simulink model "ProyectoGlobal_AyCD_Cantu_LagoTejo_OPCUA"  (R2021a)
settings: Solver=ode23  StartTime=0.0  StopTime=inf  MinStep=1e-4
values from neighbouring files (symbols this model uses):
  a_hMax = 0.75    [Datos_ProyectoGlobal_AyCD_Cantu_LagoTejo.m]    (also in Datos_v18.m; PID_calculado.mat)
  a_tMax = 0.8    [Datos_ProyectoGlobal_AyCD_Cantu_LagoTejo.m]    (also in Datos_v18.m; PID_calculado.mat)
  b_cx = 1e6    (= 1000000)    [Datos_ProyectoGlobal_AyCD_Cantu_LagoTejo.m]    (also in Datos_v18.m; PID_calculado.mat)
  b_cy = 1e7    (= 10000000)    [Datos_ProyectoGlobal_AyCD_Cantu_LagoTejo.m]    (also in Datos_v18.m; PID_calculado.mat)
  b_eq_h = ((b_hd + b_hm*(i_h^2))*2/(r_hd^2))    (= 31004.4444444)    [Datos_ProyectoGlobal_AyCD_Cantu_LagoTejo.m]    (also in Datos_v18.m; PID_calculado.mat)
  b_eq_t = ((b_td + b_tm*(i_t^2))/(r_td^2))    (= 21607.2)    [Datos_ProyectoGlobal_AyCD_Cantu_LagoTejo.m]    (also in Datos_v18.m; PID_calculado.mat)
  b_hb = 1e8    (= 100000000)    [Datos_ProyectoGlobal_AyCD_Cantu_LagoTejo.m]    (also in Datos_v18.m; PID_calculado.mat)
  b_hEb = 2.2e9    (= 2200000000)    [Datos_ProyectoGlobal_AyCD_Cantu_LagoTejo.m]    (also in Datos_v18.m; PID_calculado.mat)
  b_t = 90    [Datos_ProyectoGlobal_AyCD_Cantu_LagoTejo.m]    (also in Datos_v18.m; PID_calculado.mat)
  b_tb = 5e6    (= 5000000)    [Datos_ProyectoGlobal_AyCD_Cantu_LagoTejo.m]    (also in Datos_v18.m; PID_calculado.mat)
  b_tw = 3e3    (= 3000)    [Datos_ProyectoGlobal_AyCD_Cantu_LagoTejo.m]    (also in Datos_v18.m; PID_calculado.mat)
  b_wu = 150    [Datos_ProyectoGlobal_AyCD_Cantu_LagoTejo.m]    (also in Datos_v18.m; PID_calculado.mat)
  bah = M_eq_h*n_h*omega_h    [PID_Izaje_B.m]    (also in PID_calculado.mat = 387555.555556)
  bat = M_eq_t*n_t*omega_t    [PID_Carro_B.m]    (also in PID_calculado.mat = 270090)
  CI_h = 5    [Datos_ProyectoGlobal_AyCD_Cantu_LagoTejo.m]    (also in Datos_v18.m; PID_calculado.mat)
  CI_t = -16.25    [Datos_ProyectoGlobal_AyCD_Cantu_LagoTejo.m]    (also in Datos_v18.m; PID_calculado.mat)
  g = 9.80665    [Datos_ProyectoGlobal_AyCD_Cantu_LagoTejo.m]    (also in Datos_v18.m; PID_calculado.mat)
  H_c = 2.5    [Datos_ProyectoGlobal_AyCD_Cantu_LagoTejo.m]    (also in Datos_v18.m; PID_calculado.mat)
  i_h = 22    [Datos_ProyectoGlobal_AyCD_Cantu_LagoTejo.m]    (also in Datos_v18.m; PID_calculado.mat)
  i_t = 30    [Datos_ProyectoGlobal_AyCD_Cantu_LagoTejo.m]    (also in Datos_v18.m; PID_calculado.mat)
  k_cy = 1.8e9    (= 1800000000)    [Datos_ProyectoGlobal_AyCD_Cantu_LagoTejo.m]    (also in Datos_v18.m; PID_calculado.mat)
  k_tw = 4.8e5    (= 480000)    [Datos_ProyectoGlobal_AyCD_Cantu_LagoTejo.m]    (also in Datos_v18.m; PID_calculado.mat)
  k_wu = 2.36e8    (= 236000000)    [Datos_ProyectoGlobal_AyCD_Cantu_LagoTejo.m]    (also in Datos_v18.m; PID_calculado.mat)
  Kd_bal = [-2.22044604925e-16 2.22044604925e-16 2.22044604925e-16 0 0 0 0 0 -2.22044604925e-16 0 2.22044604925e-16 -2.22044604925e-16 ... (296091 elements, 501x591)]    [Kp_Kd_balanceo.mat]    (also in PD_Balanceo.m = zeros(length(ML),length(L)))
  Kp_bal = [5.11381136401 5.1081388039 5.10248507909 5.09685008556 5.09123372013 5.08563588037 5.08005646467 5.07449537218 5.06895250283 5.06342775732 5.05792103709 5.05243224433 ... (296091 elements, 501x591)]    [Kp_Kd_balanceo.mat]    (also in PD_Balanceo.m = Kd_bal)
  ksah = M_eq_h*n_h*(omega_h^2)    [PID_Izaje_B.m]    (also in PID_calculado.mat = 922348.374575)
  ksat = M_eq_t*n_t*(omega_t^2)    [PID_Carro_B.m]    (also in PID_calculado.mat = 972648.108)
  ksiah = M_eq_h*n_h*(omega_h^3)    [PID_Izaje_B.m]    (also in PID_calculado.mat = 2195108.57705)
  ksiat = M_eq_t*n_t*(omega_t^3)    [PID_Carro_B.m]    (also in PID_calculado.mat = 3502700.36653)
  lim_xDer = 50    [Datos_ProyectoGlobal_AyCD_Cantu_LagoTejo.m]    (also in Datos_v18.m; PID_calculado.mat)
  lim_xDer_ult = 51    [Datos_ProyectoGlobal_AyCD_Cantu_LagoTejo.m]    (also in Datos_v18.m; PID_calculado.mat)
  lim_xIzq = -30    [Datos_ProyectoGlobal_AyCD_Cantu_LagoTejo.m]    (also in Datos_v18.m; PID_calculado.mat)
  lim_xIzq_ult = -31    [Datos_ProyectoGlobal_AyCD_Cantu_LagoTejo.m]    (also in Datos_v18.m; PID_calculado.mat)
  lim_yInf = -20    [Datos_ProyectoGlobal_AyCD_Cantu_LagoTejo.m]    (also in Datos_v18.m; PID_calculado.mat)
  lim_yInf_ult = -21    [Datos_ProyectoGlobal_AyCD_Cantu_LagoTejo.m]    (also in Datos_v18.m; PID_calculado.mat)
  lim_ySup = 40    [Datos_ProyectoGlobal_AyCD_Cantu_LagoTejo.m]    (also in Datos_v18.m; PID_calculado.mat)
  lim_ySup_ult = 41    [Datos_ProyectoGlobal_AyCD_Cantu_LagoTejo.m]    (also in Datos_v18.m; PID_calculado.mat)
  M_cMax = 50000    [Datos_ProyectoGlobal_AyCD_Cantu_LagoTejo.m]    (also in Datos_v18.m; PID_calculado.mat)
  M_cMin = 2000    [Datos_ProyectoGlobal_AyCD_Cantu_LagoTejo.m]    (also in Datos_v18.m; PID_calculado.mat)
  M_eq_h = (J_hd_hEb+J_hm_hb*i_h^2)*2/r_hd^2    (= 65137.7777778)    [Datos_ProyectoGlobal_AyCD_Cantu_LagoTejo.m]    (also in Datos_v18.m; PID_calculado.mat)
  M_eq_t = ((J_td + J_tm_tb*(i_t^2))/(r_td^2))    (= 30000)    [Datos_ProyectoGlobal_AyCD_Cantu_LagoTejo.m]    (also in Datos_v18.m; PID_calculado.mat)
  M_s = 15000    [Datos_ProyectoGlobal_AyCD_Cantu_LagoTejo.m]    (also in Datos_v18.m; PID_calculado.mat)
  M_t = 30000    [Datos_ProyectoGlobal_AyCD_Cantu_LagoTejo.m]    (also in Datos_v18.m; PID_calculado.mat)
  r_hd = 0.75    [Datos_ProyectoGlobal_AyCD_Cantu_LagoTejo.m]    (also in Datos_v18.m; PID_calculado.mat)
  r_td = 0.5    [Datos_ProyectoGlobal_AyCD_Cantu_LagoTejo.m]    (also in Datos_v18.m; PID_calculado.mat)
  T_hbMax = 5e4    (= 50000)    [Datos_ProyectoGlobal_AyCD_Cantu_LagoTejo.m]    (also in Datos_v18.m; PID_calculado.mat)
  T_hEbMax = 1.1e6    (= 1100000)    [Datos_ProyectoGlobal_AyCD_Cantu_LagoTejo.m]    (also in Datos_v18.m; PID_calculado.mat)
  T_hmMax = 2e4    (= 20000)    [Datos_ProyectoGlobal_AyCD_Cantu_LagoTejo.m]    (also in Datos_v18.m; PID_calculado.mat)
  T_tbMax = 5e3    (= 5000)    [Datos_ProyectoGlobal_AyCD_Cantu_LagoTejo.m]    (also in Datos_v18.m; PID_calculado.mat)
  T_tmMax = 3e3    (= 3000)    [Datos_ProyectoGlobal_AyCD_Cantu_LagoTejo.m]    (also in Datos_v18.m; PID_calculado.mat)
  tau_hm = 1e-3    (= 0.001)    [Datos_ProyectoGlobal_AyCD_Cantu_LagoTejo.m]    (also in Datos_v18.m; PID_calculado.mat)
  tau_tm = 1e-3    (= 0.001)    [Datos_ProyectoGlobal_AyCD_Cantu_LagoTejo.m]    (also in Datos_v18.m; PID_calculado.mat)
  v_hMax_0 = 3    [Datos_ProyectoGlobal_AyCD_Cantu_LagoTejo.m]    (also in Datos_v18.m; PID_calculado.mat)
  v_tMax = 4    [Datos_ProyectoGlobal_AyCD_Cantu_LagoTejo.m]    (also in Datos_v18.m; PID_calculado.mat)
  xc = [-28.75 -26.25 -23.75 -21.25 -18.75 -16.25 -13.75 -11.25 -8.75 -6.25 -3.75 -1.25 ... (32 elements, 1x32)]    [PID_calculado.mat]    (also in Perfil_Carga.m = -30+1.25:2.5:50-1.25)
  Y_t0 = 45    [Datos_ProyectoGlobal_AyCD_Cantu_LagoTejo.m]    (also in Datos_v18.m; PID_calculado.mat)
  yc = [0 0 0 2.5 0 2.5 0 2.5 0 0 0 0 ... (32 elements, 1x32)]    [PID_calculado.mat]    (also in Perfil_Carga.m = yc2)
undefined symbols (not defined in the file or in its folder): bcx, bcy, Cond_Ini_h, Cond_Ini_t, Kcy
libraries: simulink x13, opclib x3
(part 1 of 3)
settings Model: SimulationMode=accelerator  Creator=Maxi  LastModifiedBy=maxim
settings SolverCC: InitialStep=1e-3  MaxConsecutiveZCs=10000  MaxConsecutiveMinStep=10000000  ZeroCrossAlgorithm=Adaptive  AlgebraicLoopSolver=TrustRegion
settings DebuggingCC: AlgebraicLoopMsg=none  MaskedZcDiagnostic=none  IgnoredZcDiagnostic=none  SFUnusedDataAndEventsDiag=none  UnderSpecifiedDimensionMsg=warning
settings RTWCC: DLArmComputeVersion=20.02.1

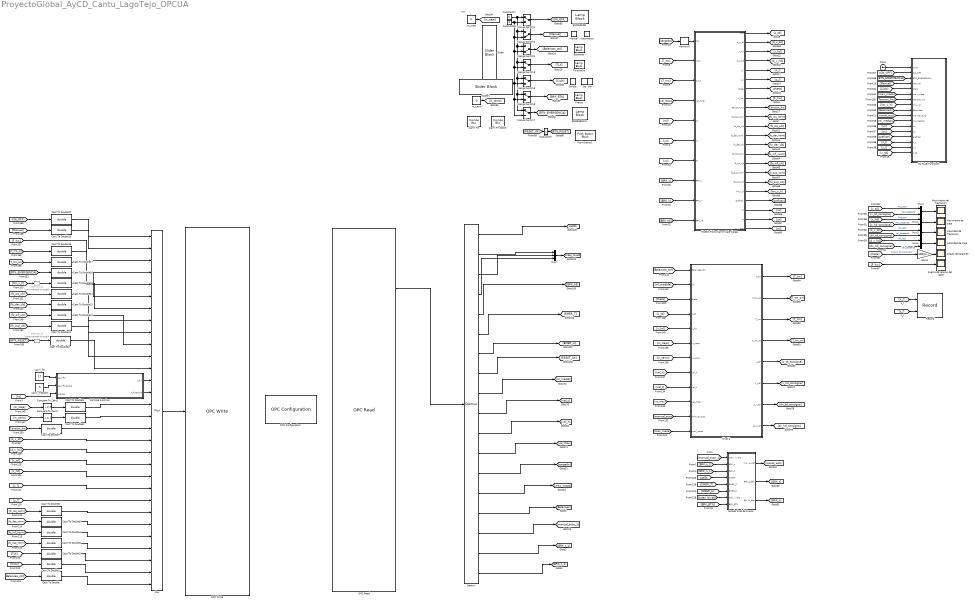
== system ProyectoGlobal_AyCD_Cantu_LagoTejo_OPCUA ==
  note: HMI
  "  Do" : LampBlock  LabelPosition=Hide
  Angulo de balanceo : Scope
  Automático : LampBlock  LabelPosition=Hide
  Balanceo : LampBlock  LabelPosition=Hide
  Carril Fin : ComboBox  LabelPosition=Hide  SelectedLabel=17
      settings: Values={{'1', '2', '3', '4', '5', '6', '7', '8', '9', '10', '11', '12', '13', '14', '15', '16', '17', '18'}, [1 2 3 4 5 6 7 8 9 10 11 12 13 14 15 16 17 18]}
  Carril Fin Doble : ComboBox  LabelPosition=Hide  SelectedLabel=5
      settings: Values={{'1', '2', '3', '4', '5', '6', '7', '8', '9', '10', '11', '12', '13', '14', '15', '16', '17', '18'}, [1 2 3 4 5 6 7 8 9 10 11 12 13 14 15 16 17 18]}
  Cast To Double{,1..20} (21 alike) : DataTypeConversion  OutDataTypeStr=double
  Clock : Clock
  Compare To Zero2 : simulink/Logic and Bit Operations/Compare To Zero  relop=~=  OutDataTypeStr=boolean
  Compare To Zero7 : simulink/Logic and Bit Operations/Compare To Zero  relop=~=  OutDataTypeStr=boolean
  Constant17 : Constant  Value=0
  Constant18 : Constant
  Demux : Demux  Outputs=18
  EMERGENCIA : LampBlock  LabelPosition=Hide
  ENCENDIDO : LampBlock  LabelPosition=Hide
  Estado Final de Frenos : Subsystem
  Frenos : LampBlock  LabelPosition=Hide
  Fuerza de tension del cable : Scope
  Gain3 : Gain  Gain=180/pi
  MATLAB Function : MATLAB Function  TreatAsAtomicUnit=on
  MATLAB Function1 : MATLAB Function  TreatAsAtomicUnit=on
  Manual : LampBlock  LabelPosition=Hide
  Manual Switch{1,3,5..7} (5 alike) : ManualSwitch
  Manual Switch2 : ManualSwitch  CurrentSetting=0
  Manual Switch4 : ManualSwitch  CurrentSetting=0
  Memory10 : Memory  Commented=through
  Memory12 : Memory  Commented=through
  Memory5 : Memory
  Modelo Fisico Carro-Izaje-Carga : Subsystem
  Movimiento de Izaje : Scope
  Movimiento de Traslacion : Scope
  Mux : Mux  Inputs=30
  Mux{1..4} (4 alike) : Mux  Inputs=2
  Mux7 : Mux  Inputs=3
  Nivel 2 : Subsystem
  OPC Configuration : opclib/OPC Configuration  opcServers=localhost/CoDeSys.OPC.DA/10  errMissingItems=Error  errReadWrite=Warn  errShutdown=Error  errRTViolation=Warn  rtEnable=on  speedup=1  showLatency=off  beingUsed=on
      settings: SourceProductBaseCode=OT
  OPC Read : opclib/OPC Read  serverHost=localhost  serverID=CoDeSys.OPC.DA  itemIDs=PLC1.Application.GVL.sistOK, PLC1.Application.GVL.manual_auto_N0, PLC1.Application.GVL.BRK_t_N0, PLC1.Application.GVL.BRK_h_N0, PLC1.Application.GVL.BRK_hE, PLC1.Application.GVL.EMER_t, PLC1.Application.GVL.EMER_h, PLC1.Application.GVL.RESET_OK, PLC1.Application.GVL.m_l_calc, PLC1.Application.GVL.vel_t, PLC1.Application.GVL.vel_h, PLC1.Application.GVL.vel_hMax, PLC1.Application.GVL.cargado, PLC1.Application.GVL.max_masa, PLC1.Application.GVL.Balanceo, PLC1.Application.GVL.manual_auto_N1, PLC1.Application.GVL.BRK_t_N1, PLC1.Application.GVL.BRK_h_N1  readMode=Synchronous (cache)  dataType=double  updateRate=0.5  showQual=on  showTS=on  tsMode=Seconds since start
      settings: SourceProductBaseCode=OT
  OPC Write : opclib/OPC Write  serverHost=localhost  serverID=CoDeSys.OPC.DA  itemIDs=PLC1.Application.GVL.ON_OFF, PLC1.Application.GVL.Manual, PLC1.Application.GVL.F_hw, PLC1.Application.GVL.T_hm_on, PLC1.Application.GVL.T_tm_on, PLC1.Application.GVL.BTN_EMERGENCIA, PLC1.Application.GVL.lim_v_h, PLC1.Application.GVL.fc_izq_ult, PLC1.Application.GVL.fc_der_ult, PLC1.Application.GVL.fc_inf_ult, PLC1.Application.GVL.fc_sup_ult, PLC1.Application.GVL.BTN_RESET, PLC1.Application.GVL.X_fin, PLC1.Application.GVL.X_finDoble, PLC1.Application.GVL.in_izaje_on, PLC1.Application.GVL.in_carro_on, PLC1.Application.GVL.Tension_hw, PLC1.Application.GVL.d_x_td, PLC1.Application.GVL.d_x_h, PLC1.Application.GVL.x_td, PLC1.Application.GVL.x_h, PLC1.Application.GVL.x_l, PLC1.Application.GVL.y_l, PLC1.Application.GVL.fc_izq_norm, PLC1.Application.GVL.fc_der_norm, PLC1.Application.GVL.fc_inf_norm, PLC1.Application.GVL.fc_sup_norm, PLC1.Application.GVL.TLK, PLC1.Application.GVL.Ciclo_Doble, PLC1.Application.GVL.Balanceo_ctrl  writeMode=Synchronous  updateRate=0
      settings: SourceProductBaseCode=OT
  Push Button1 : PushButtonBlock  ButtonText=RESET
  Record : Record  FileSettingsInternal="{\"entries\":[{\"content\":{\"excelSettings\":{\"content\":{},\"type\":\"Streamout.ExcelSettings\"}},\"type\":\"Streamout.FileSettingStorage\",\"uuid\":\"560a1c1a-7c8f-45a0-acac-2ad7503fa280\"}],\"packageUris\":[\"http://schema.mathworks.com/mf0/streamout_blocks/R2020a\"],\"version\":\"1.0\"}"  Layout=[1 1]  SignalsInternal="{\"entries\":[{\"content\":{\"signals\":[{\"content\":{\"blockPath\":[\"modelo_fisico_OPCUA/Record\"],\"channel\":[],\"dimensions\":[1],\"domain\":\"modelo_fisico_opcua/record\",\"lineColor\":\"#edb120\",\"plots\":[1],\"port\":1,\"sid\":[],\"signalID\":9,\"signalName\":\"x_l\"},\"type\":\"RecordBlkView.Signal\",\"uuid\":\"8ed411c4-7e14-4ae8-9e7a-a46f1e662131\"},{\"content\":{\"blockPath\":[\"modelo_fisico_OPCUA/Record\"],\"channel\":[],\"dimensions\":[1],\"domain\":\"modelo_fisico_opcua/record\",\"lineColor\":\"#7e2f8e\",\"plots\":[1],\"port\":2,\"sid\":[],\"signalID\":12,\"signalName\":\"y_l\"},\"type\":\"RecordBlkView.Signal\",\"uuid\":\"8d6d7a06-d56f-446f-a3f9-26de8d86f7e4\"},{\"content\":{\"blockPath\":[\"modelo_fisico_OPCUA/Record\"],\"channel\":[],\"dimensions\":[1,32],\"domain\":\"modelo_fisico_opcua/record\",\"hasChildren\":true,\"lineColor\":\"#77ac30\",\"plots\":[],\"port\":3,\"sid\":[],\"signalID\":15,\"signalName\":\"x_perfil\"},\"type\":\"RecordBlkView.Signal\",\"uuid\":\"b525593d-bc80-4908-881a-e4ffaca2af93\"},{\"content\":{\"blockPath\":[\"modelo_fisico_OPCUA/Record\"],\"channel\":[1,1],\"dimensions\":[1,32],\"domain\":\"modelo_fisico_opcua/record\",\"lineColor\":\"#4dbeee\",\"parentID\":15,\"plots\":[1],\"port\":3,\"sid\":[],\"signalID\":16,\"signalName\":\"x_perfil\"},\"type\":\"RecordBlkView.Signal\",\"uuid\":\"6a90bcad-4de9-4ccf-acf1-2125847e7892\"},{\"content\":{\"blockPath\":[\"modelo_fisico_OPCUA/Record\"],\"channel\":[1,2],\"dimensions\":[1,32],\"domain\":\"modelo_fisico_opcua/record\",\"lineColor\":\"#fe330a\",\"parentID\":15,\"plots\":[1],\"port\":3,\"sid\":[],\"signalID\":17,\"signalName\":\"x_perfil\"},\"type\":\"RecordBlkView.Signal\",\"uuid\":\"817aff20-781c-415f-a325-38912855be13\"},{\"content\":{\"blockPath\":[\"modelo_fisico_OPCUA/Record\"],\"channel\":[1,3],\"dimensions\":[1,32],\"domain\":\"modelo_fisico_opcua/record\",\"lineColor\":\"#22b573\",\"parentID\":15,\"plots\":[],\"port\":3,\"sid\":[],\"signalID\":18,\"signalName\":\"x_perfil\"},\"type\":\"RecordBlkView.Signal\",\"uuid\":\"17ad2ace-c9b0-4e9e-99ad-e43776de256b\"},{\"content\":{\"blockPath\":[\"modelo_fisico_OPCUA/Record\"],\"channel\":[1,4],\"dimensions\":[1,32],\"domain\":\"modelo_fisico_opcua/record\",\"lineColor\":\"#0072bd\",\"parentID\":15,\"plots\":[],\"port\":3,\"sid\":[],\"signalID\":19,\"signalName\":\"x_perfil\"},\"type\":\"RecordBlkView.Signal\",\"uuid\":\"ac0c197e-63a8-4e14-82ce-1afe2d8e9646\"},{\"content\":{\"blockPath\":[\"modelo_fisico_OPCUA/Record\"],\"channel\":[1,5],\"dimensions\":[1,32],\"domain\":\"modelo_fisico_opcua/record\",\"lineColor\":\"#d95319\",\"parentID\":15,\"plots\":[],\"port\":3,\"sid\":[],\"signalID\":20,\"signalName\":\"x_perfil\"},\"type\":\"RecordBlkView.Signal\",\"uuid\":\"b2dea709-1f7a-42de-b271-3351a57e50b4\"},{\"content\":{\"blockPath\":[\"modelo_fisico_OPCUA/Record\"],\"channel\":[1,6],\"dimensions\":[1,32],\"domain\":\"modelo_fisico_opcua/record\",\"lineColor\":\"#edb120\",\"parentID\":15,\"plots\":[],\"port\":3,\"sid\":[],\"signalID\":21,\"signalName\":\"x_perfil\"},\"type\":\"RecordBlkView.Signal\",\"uuid\":\"7040c539-c6c4-468b-b363-9105d925f59a\"},{\"content\":{\"blockPath\":[\"modelo_fisico_OPCUA/Record\"],\"channel\":[1,7],\"dimensions\":[1,32],\"domain\":\"modelo_fisico_opcua/record\",\"lineColor\":\"#7e2f8e\",\"parentID\":15,\"plots\":[],\"port\":3,\"sid\":[],\"signalID\":22,\"signalName\":\"x_perfil\"},\"type\":\"RecordBlkView.Signal\",\"uuid\":\"838ba2aa-2cf7-44e4-98a5-f5b176c14505\"},{\"content\":{\"blockPath\":[\"modelo_fisico_OPCUA/Record\"],\"channel\":[1,8],\"dimensions\":[1,32],\"domain\":\"modelo_fisico_opcua/record\",\"lineColor\":\"#77ac30\",\"parentID\":15,\"plots\":[],\"port\":3,\"sid\":[],\"signalID\":23,\"signalName\":\"x_perfil\"},\"type\":\"RecordBlkView.Signal\",\"uuid\":\"7f7327bd-a800-48a1-ae70-9791c063e958\"},{\"content\":{\"blockPath\":[\"modelo_fisico_OPCUA/Record\"],\"channel\":[1,9],\"dimensions\":[1,32],\"domain\":\"modelo_fisico_opcua/record\",\"lineColor\":\"#4dbeee\",\"parentID\":15,\"plots\":[],\"port\":3,\"sid\":[],\"signalID\":24,\"signalName\":\"x_perfil\"},\"type\":\"RecordBlkView.Signal\",\"uuid\":\"dc46df26-7320-47c5-a126-b064752e732b\"},{\"content\":{\"blockPath\":[\"modelo_fisico_OPCUA/Record\"],\"channel\":[1,10],\"dimensions\":[1,32],\"domain\":\"modelo_fisico_opcua/record\",\"lineColor\":\"#a2142f\",\"parentID\":15,\"plots\":[],\"port\":3,\"sid\":[],\"signalID\":25,\"signalName\":\"x_perfil\"},\"type\":\"RecordBlkView.Signal\",\"uuid\":\"56351981-dee7-481d-8877-4b0a4513273c\"},{\"content\":{\"blockPath\":[\"modelo_fisico_OPCUA/Record\"],\"channel\":[1,11],\"dimensions\":[1,32],\"domain\":\"modelo_fisico_opcua/record\",\"lineColor\":\"#139fff\",\"parentID\":15,\"plots\":[],\"port\":3,\"sid\":[],\"signalID\":26,\"signalName\":\"x_perfil\"},\"type\":\"RecordBlkView.Signal\",\"uuid\":\"c3cdab0a-47b4-4906-b085-8a2ff7353c31\"},{\"content\":{\"blockPath\":[\"modelo_fisico_OPCUA/Record\"],\"channel\":[1,12],\"dimensions\":[1,32],\"domain\":\"modelo_fisico_opcua/record\",\"lineColor\":\"#ff6929\",\"parentID\":15,\"plots\":[],\"port\":3,\"sid\":[],\"signalID\":27,\"signalName\":\"x_perfil\"},\"type\":\"RecordBlkView.Signal\",\"uuid\":\"92a94ddb-972e-4b54-aa74-364505e8725e\"},{\"content\":{\"blockPath\":[\"modelo_fisico_OPCUA/Record\"],\"channel\":[1,13],\"dimensions\":[1,32],\"domain\":\"modelo_fisico_opcua/record\",\"lineColor\":\"#b746ff\",\"parentID\":15,\"plots\":[],\"port\":3,\"sid\":[],\"signalID\":28,\"signalName\":\"x_perfil\"},\"type\":\"RecordBlkView.Signal\",\"uuid\":\"cd68ec88-6bbf-4001-a489-b4ac27c14d6a\"},{\"content\":{\"blockPath\":[\"modelo_fisico_OPCUA/Record\"],\"channel\":[1,14],\"dimensions\":[1,32],\"domain\":\"modelo_fisico_opcua/record\",\"lineColor\":\"#64d413\",\"parentID\":15,\"plots\":[],\"port\":3,\"sid\":[],\"signalID\":29,\"signalName\":\"x_perfil\"},\"type\":\"RecordBlkView.Signal\",\"uuid\":\"b6b0c035-5c4a-41dd-b6ed-91ecd091e6ef\"},{\"content\":{\"blockPath\":[\"modelo_fisico_OPCUA/Record\"],\"channel\":[1,15],\"dimensions\":[1,32],\"domain\":\"modelo_fisico_opcua/record\",\"lineColor\":\"#ff13a6\",\"parentID\":15,\"plots\":[],\"port\":3,\"sid\":[],\"signalID\":30,\"signalName\":\"x_perfil\"},\"type\":\"RecordBlkView.Signal\",\"uuid\":\"61be6124-0d23-485a-9b0c-6e628ce1c532\"},{\"content\":{\"blockPath\":[\"modelo_fisico_OPCUA/Record\"],\"channel\":[1,16],\"dimensions\":[1,32],\"domain\":\"modelo_fisico_opcua/record\",\"lineColor\":\"#fe330a\",\"parentID\":15,\"plots\":[],\"port\":3,\"sid\":[],\"signalID\":31,\"signalName\":\"x_perfil\"},\"type\":\"RecordBlkView.Signal\",\"uuid\":\"78409dcb-59a0-4571-a5b6-4d7693be06be\"},{\"content\":{\"blockPath\":[\"modelo_fisico_OPCUA/Record\"],\"channel\":[1,17],\"dimensions\":[1,32],\"domain\":\"modelo_fisico_opcua/record\",\"lineColor\":\"#22b573\",\"parentID\":15,\"plots\":[],\"port\":3,\"sid\":[],\"signalID\":32,\"signalName\":\"x_perfil\"},\"type\":\"RecordBlkView.Signal\",\"uuid\":\"40228b64-1439-4b88-8512-2e6e5e0a084f\"},{\"content\":{\"blockPath\":[\"modelo_fisico_OPCUA/Record\"],\"channel\":[1,18],\"dimensions\":[1,32],\"domain\":\"modelo_fisico_opcua/record\",\"lineColor\":\"#0072bd\",\"parentID\":15,\"plots\":[],\"port\":3,\"sid\":[],\"signalID\":33,\"signalName\":\"x_perfil\"},\"type\":\"RecordBlkView.Signal\",\"uuid\":\"d580995b-d659-4183-9c4a-5b8531b5410a\"},{\"content\":{\"blockPath\":[\"modelo_fisico_OPCUA/Record\"],\"channel\":[1,19],\"dimensions\":[1,32],\"domain\":\"modelo_fisico_opcua/record\",\"lineColor\":\"#d95319\",\"parentID\":15,\"plots\":[],\"port\":3,\"sid\":[],\"signalID\":34,\"signalName\":\"x_perfil\"},\"type\":\"RecordBlkView.Signal\",\"uuid\":\"362f2464-1207-4e23-923f-332f7297835c\"},{\"content\":{\"blockPath\":[\"modelo_fisico_OPCUA/Record\"],\"channel\":[1,20],\"dimensions\":[1,32],\"domain\":\"modelo_fisico_opcua/record\",\"lineColor\":\"#edb120\",\"parentID\":15,\"plots\":[],\"port\":3,\"sid\":[],\"signalID\":35,\"signalName\":\"x_perfil\"},\"type\":\"RecordBlkView.Signal\",\"uuid\":\"1b656f07-a23b-47d3-97d5-81b48fe59d30\"},{\"content\":{\"blockPath\":[\"modelo_fisico_OPCUA/Record\"],\"channel\":[1,21],\"dimensions\":[1,32],\"domain\":\"modelo_fisico_opcua/record\",\"lineColor\":\"#7e2f8e\",\"parentID\":15,\"plots\":[],\"port\":3,\"sid\":[],\"signalID\":36,\"signalName\":\"x_perfil\"},\"type\":\"RecordBlkView.Signal\",\"uuid\":\"41f2abfa-2a9f-43c7-8411-4d69c8cedf76\"},{\"content\":{\"blockPath\":[\"modelo_fisico_OPCUA/Record\"],\"channel\":[1,22],\"dimensions\":[1,32],\"domain\":\"modelo_fisico_opcua/record\",\"lineColor\":\"#77ac30\",\"parentID\":15,\"plots\":[],\"port\":3,\"sid\":[],\"signalID\":37,\"signalName\":\"x_perfil\"},\"type\":\"RecordBlkView.Signal\",\"uuid\":\"d0094ba1-20f3-4752-91cc-c8d7dc6f31e0\"},{\"content\":{\"blockPath\":[\"modelo_fisico_OPCUA/Record\"],\"channel\":[1,23],\"dimensions\":[1,32],\"domain\":\"modelo_fisico_opcua/record\",\"lineColor\":\"#4dbeee\",\"parentID\":15,\"plots\":[],\"port\":3,\"sid\":[],\"signalID\":38,\"signalName\":\"x_perfil\"},\"type\":\"RecordBlkView.Signal\",\"uuid\":\"7f1cb14b-d968-4eae-ae96-2eef0dcef1d2\"},{\"content\":{\"blockPath\":[\"modelo_fisico_OPCUA/Record\"],\"channel\":[1,24],\"dimensions\":[1,32],\"domain\":\"modelo_fisico_opcua/record\",\"lineColor\":\"#a2142f\",\"parentID\":15,\"plots\":[],\"port\":3,\"sid\":[],\"signalID\":39,\"signalName\":\"x_perfil\"},\"type\":\"RecordBlkView.Signal\",\"uuid\":\"a149b9b0-469b-4dee-b6a3-c3848182e778\"},{\"content\":{\"blockPath\":[\"modelo_fisico_OPCUA/Record\"],\"channel\":[1,25],\"dimensions\":[1,32],\"domain\":\"modelo_fisico_opcua/record\",\"lineColor\":\"#139fff\",\"parentID\":15,\"plots\":[],\"port\":3,\"sid\":[],\"signalID\":40,\"signalName\":\"x_perfil\"},\"type\":\"RecordBlkView.Signal\",\"uuid\":\"d2acd9f4-bf56-4995-9e9d-05fcbf398416\"},{\"content\":{\"blockPath\":[\"modelo_fisico_OPCUA/Record\"],\"channel\":[1,26],\"dimensions\":[1,32],\"domain\":\"modelo_fisico_opcua/record\",\"lineColor\":\"#ff6929\",\"parentID\":15,\"plots\":[],\"port\":3,\"sid\":[],\"signalID\":41,\"signalName\":\"x_perfil\"},\"type\":\"RecordBlkView.Signal\",\"uuid\":\"ec458ff0-2fe1-4e87-80ed-b9e014563081\"},{\"content\":{\"blockPath\":[\"modelo_fisico_OPCUA/Record\"],\"channel\":[1,27],\"dimensions\":[1,32],\"domain\":\"modelo_fisico_opcua/record\",\"lineColor\":\"#b746ff\",\"parentID\":15,\"plots\":[],\"port\":3,\"sid\":[],\"signalID\":42,\"signalName\":\"x_perfil\"},\"type\":\"RecordBlkView.Signal\",\"uuid\":\"6100f097-16d9-4f59-a052-147391a280cc\"},{\"content\":{\"blockPath\":[\"modelo_fisico_OPCUA/Record\"],\"channel\":[1,28],\"dimensions\":[1,32],\"domain\":\"modelo_fisico_opcua/record\",\"lineColor\":\"#64d413\",\"parentID\":15,\"plots\":[],\"port\":3,\"sid\":[],\"signalID\":43,\"signalName\":\"x_perfil\"},\"type\":\"RecordBlkView.Signal\",\"uuid\":\"f8afc42e-bebd-45e5-8773-ff8c2b40aedf\"},{\"content\":{\"blockPath\":[\"modelo_fisico_OPCUA/Record\"],\"channel\":[1,29],\"dimensions\":[1,32],\"domain\":\"modelo_fisico_opcua/record\",\"lineColor\":\"#ff13a6\",\"parentID\":15,\"plots\":[],\"port\":3,\"sid\":[],\"signalID\":44,\"signalName\":\"x_perfil\"},\"type\":\"RecordBlkView.Signal\",\"uuid\":\"3812678c-63e2-494a-8659-62fc09d91819\"},{\"content\":{\"blockPath\":[\"modelo_fisico_OPCUA/Record\"],\"channel\":[1,30],\"dimensions\":[1,32],\"domain\":\"modelo_fisico_opcua/record\",\"lineColor\":\"#fe330a\",\"parentID\":15,\"plots\":[],\"port\":3,\"sid\":[],\"signalID\":45,\"signalName\":\"x_perfil\"},\"type\":\"RecordBlkView.Signal\",\"uuid\":\"d3c92ddf-bef8-4ed9-8d40-50167eef2e7e\"},{\"content\":{\"blockPath\":[\"modelo_fisico_OPCUA/Record\"],\"channel\":[1,31],\"dimensions\":[1,32],\"domain\":\"modelo_fisico_opcua/record\",\"lineColor\":\"#22b573\",\"parentID\":15,\"plots\":[],\"port\":3,\"sid\":[],\"signalID\":46,\"signalName\":\"x_perfil\"},\"type\":\"RecordBlkView.Signal\",\"uuid\":\"6d648390-cc78-4833-a260-807b7828dc8a\"},{\"content\":{\"blockPath\":[\"modelo_fisico_OPCUA/Record\"],\"channel\":[1,32],\"dimensions\":[1,32],\"domain\":\"modelo_fisico_opcua/record\",\"lineColor\":\"#0072bd\",\"parentID\":15,\"plots\":[],\"port\":3,\"sid\":[],\"signalID\":47,\"signalName\":\"x_perfil\"},\"type\":\"RecordBlkView.Signal\",\"uuid\":\"42ae7673-7115-413a-868b-999b1065caa5\"},{\"content\":{\"blockPath\":[\"modelo_fisico_OPCUA/Record\"],\"channel\":[],\"dimensions\":[1,32],\"domain\":\"modelo_fisico_opcua/record\",\"hasChildren\":true,\"lineColor\":\"#a2142f\",\"plots\":[],\"port\":4,\"sid\":[],\"signalID\":82,\"signalName\":\"y_perfil\"},\"type\":\"RecordBlkView.Signal\",\"uuid\":\"d9f90962-6edd-4ec0-abe8-dd100a7f8a50\"},{\"content\":{\"blockPath\":[\"modelo_fisico_OPCUA/Record\"],\"channel\":[1,1],\"dimensions\":[1,32],\"domain\":\"modelo_fisico_opcua/record\",\"lineColor\":\"#139fff\",\"parentID\":82,\"plots\":[1],\"port\":4,\"sid\":[],\"signalID\":83,\"signalName\":\"y_perfil\"},\"type\":\"RecordBlkView.Signal\",\"uuid\":\"06b64a56-2c15-4519-8c10-7e671d1ef7ae\"},{\"content\":{\"blockPath\":[\"modelo_fisico_OPCUA/Record\"],\"channel\":[1,2],\"dimensions\":[1,32],\"domain\":\"modelo_fisico_opcua/record\",\"lineColor\":\"#d95319\",\"parentID\":82,\"plots\":[1],\"port\":4,\"sid\":[],\"signalID\":84,\"signalName\":\"y_perfil\"},\"type\":\"RecordBlkView.Signal\",\"uuid\":\"5fbd3c29-b525-4d08-ad80-dda292280f2b\"},{\"content\":{\"blockPath\":[\"modelo_fisico_OPCUA/Record\"],\"channel\":[1,3],\"dimensions\":[1,32],\"domain\":\"modelo_fisico_opcua/record\",\"lineColor\":\"#edb120\",\"parentID\":82,\"plots\":[],\"port\":4,\"sid\":[],\"signalID\":85,\"signalName\":\"y_perfil\"},\"type\":\"RecordBlkView.Signal\",\"uuid\":\"9489a3ba-12fc-47aa-bb2b-982bf65acc83\"},{\"content\":{\"blockPath\":[\"modelo_fisico_OPCUA/Record\"],\"channel\":[1,4],\"dimensions\":[1,32],\"domain\":\"modelo_fisico_opcua/record\",\"lineColor\":\"#7e2f8e\",\"parentID\":82,\"plots\":[],\"port\":4,\"sid\":[],\"signalID\":86,\"signalName\":\"y_perfil\"},\"type\":\"RecordBlkView.Signal\",\"uuid\":\"12117092-dea8-4a8e-a8b8-5264225c9133\"},{\"content\":{\"blockPath\":[\"modelo_fisico_OPCUA/Record\"],\"channel\":[1,5],\"dimensions\":[1,32],\"domain\":\"modelo_fisico_opcua/record\",\"lineColor\":\"#77ac30\",\"parentID\":82,\"plots\":[],\"port\":4,\"sid\":[],\"signalID\":87,\"signalName\":\"y_perfil\"},\"type\":\"RecordBlkView.Signal\",\"uuid\":\"3b763b01-e259-46f7-a043-73c60a8d4745\"},{\"content\":{\"blockPath\":[\"modelo_fisico_OPCUA/Record\"],\"channel\":[1,6],\"dimensions\":[1,32],\"domain\":\"modelo_fisico_opcua/record\",\"lineColor\":\"#4dbeee\",\"parentID\":82,\"plots\":[],\"port\":4,\"sid\":[],\"signalID\":88,\"signalName\":\"y_perfil\"},\"type\":\"RecordBlkView.Signal\",\"uuid\":\"3962a667-a6fe-4be6-9a61-c4fbe910ef5f\"},{\"content\":{\"blockPath\":[\"modelo_fisico_OPCUA/Record\"],\"channel\":[1,7],\"dimensions\":[1,32],\"domain\":\"modelo_fisico_opcua/record\",\"lineColor\":\"#a2142f\",\"parentID\":82,\"plots\":[],\"port\":4,\"sid\":[],\"signalID\":89,\"signalName\":\"y_perfil\"},\"type\":\"RecordBlkView.Signal\",\"uuid\":\"f27eb6c0-2ddc-4c38-a834-ebc399d71a7c\"},{\"content\":{\"blockPath\":[\"modelo_fisico_OPCUA/Record\"],\"channel\":[1,8],\"dimensions\":[1,32],\"domain\":\"modelo_fisico_opcua/record\",\"lineColor\":\"#139fff\",\"parentID\":82,\"plots\":[],\"port\":4,\"sid\":[],\"signalID\":90,\"signalName\":\"y_perfil\"},\"type\":\"RecordBlkView.Signal\",\"uuid\":\"c3f39b4b-3486-47ed-86bd-34da47593f3c\"},{\"content\":{\"blockPath\":[\"modelo_fisico_OPCUA/Record\"],\"channel\":[1,9],\"dimensions\":[1,32],\"domain\":\"modelo_fisico_opcua/record\",\"lineColor\":\"#ff6929\",\"parentID\":82,\"plots\":[],\"port\":4,\"sid\":[],\"signalID\":91,\"signalName\":\"y_perfil\"},\"type\":\"RecordBlkView.Signal\",\"uuid\":\"c598072b-d90f-4b6b-861e-e53c3de91533\"},{\"content\":{\"blockPath\":[\"modelo_fisico_OPCUA/Record\"],\"channel\":[1,10],\"dimensions\":[1,32],\"domain\":\"modelo_fisico_opcua/record\",\"lineColor\":\"#b746ff\",\"parentID\":82,\"plots\":[],\"port\":4,\"sid\":[],\"signalID\":92,\"signalName\":\"y_perfil\"},\"type\":\"RecordBlkView.Signal\",\"uuid\":\"2f3810d4-798f-48a7-bd67-4647fc5c2990\"},{\"content\":{\"blockPath\":[\"modelo_fisico_OPCUA/Record\"],\"channel\":[1,11],\"dimensions\":[1,32],\"domain\":\"modelo_fisico_opcua/record\",\"lineColor\":\"#64d413\",\"parentID\":82,\"plots\":[],\"port\":4,\"sid\":[],\"signalID\":93,\"signalName\":\"y_perfil\"},\"type\":\"RecordBlkView.Signal\",\"uuid\":\"c0af05f3-4e0f-441e-936b-860e4cc07fd4\"},{\"content\":{\"blockPath\":[\"modelo_fisico_OPCUA/Record\"],\"channel\":[1,12],\"dimensions\":[1,32],\"domain\":\"modelo_fisico_opcua/record\",\"lineColor\":\"#ff13a6\",\"parentID\":82,\"plots\":[],\"port\":4,\"sid\":[],\"signalID\":94,\"signalName\":\"y_perfil\"},\"type\":\"RecordBlkView.Signal\",\"uuid\":\"88dd4e19-5e1b-4e4e-a2b7-42439597bb32\"},{\"content\":{\"blockPath\":[\"modelo_fisico_OPCUA/Record\"],\"channel\":[1,13],\"dimensions\":[1,32],\"domain\":\"modelo_fisico_opcua/record\",\"lineColor\":\"#fe330a\",\"parentID\":82,\"plots\":[],\"port\":4,\"sid\":[],\"signalID\":95,\"signalName\":\"y_perfil\"},\"type\":\"RecordBlkView.Signal\",\"uuid\":\"472950a7-6a04-4c18-80e7-ec17a3b9bdd0\"},{\"content\":{\"blockPath\":[\"modelo_fisico_OPCUA/Record\"],\"channel\":[1,14],\"dimensions\":[1,32],\"domain\":\"modelo_fisico_opcua/record\",\"lineColor\":\"#22b573\",\"parentID\":82,\"plots\":[],\"port\":4,\"sid\":[],\"signalID\":96,\"signalName\":\"y_perfil\"},\"type\":\"RecordBlkView.Signal\",\"uuid\":\"b184d62d-1ce3-431c-818b-dfbc37fdbd4b\"},{\"content\":{\"blockPath\":[\"modelo_fisico_OPCUA/Record\"],\"channel\":[1,15],\"dimensions\":[1,32],\"domain\":\"modelo_fisico_opcua/record\",\"lineColor\":\"#0072bd\",\"parentID\":82,\"plots\":[],\"port\":4,\"sid\":[],\"signalID\":97,\"signalName\":\"y_perfil\"},\"type\":\"RecordBlkView.Signal\",\"uuid\":\"0fc82469-3e7a-4fd0-b72c-a38c6d423a6c\"},{\"content\":{\"blockPath\":[\"modelo_fisico_OPCUA/Record\"],\"channel\":[1,16],\"dimensions\":[1,32],\"domain\":\"modelo_fisico_opcua/record\",\"lineColor\":\"#d95319\",\"parentID\":82,\"plots\":[],\"port\":4,\"sid\":[],\"signalID\":98,\"signalName\":\"y_perfil\"},\"type\":\"RecordBlkView.Signal\",\"uuid\":\"26e3f7df-eb6c-47a6-ab40-ed8246f77387\"},{\"content\":{\"blockPath\":[\"modelo_fisico_OPCUA/Record\"],\"channel\":[1,17],\"dimensions\":[1,32],\"domain\":\"modelo_fisico_opcua/record\",\"lineColor\":\"#edb120\",\"parentID\":82,\"plots\":[],\"port\":4,\"sid\":[],\"signalID\":99,\"signalName\":\"y_perfil\"},\"type\":\"RecordBlkView.Signal\",\"uuid\":\"6c2c651d-418c-4fad-9cdc-7fdd0a0661a9\"},{\"content\":{\"blockPath\":[\"modelo_fisico_OPCUA/Record\"],\"channel\":[1,18],\"dimensions\":[1,32],\"domain\":\"modelo_fisico_opcua/record\",\"lineColor\":\"#7e2f8e\",\"parentID\":82,\"plots\":[],\"port\":4,\"sid\":[],\"signalID\":100,\"signalName\":\"y_perfil\"},\"type\":\"RecordBlkView.Signal\",\"uuid\":\"39474529-1a78-4fea-8b0b-9c9e9ee94a7e\"},{\"content\":{\"blockPath\":[\"modelo_fisico_OPCUA/Record\"],\"channel\":[1,19],\"dimensions\":[1,32],\"domain\":\"modelo_fisico_opcua/record\",\"lineColor\":\"#77ac30\",\"parentID\":82,\"plots\":[],\"port\":4,\"sid\":[],\"signalID\":101,\"signalName\":\"y_perfil\"},\"type\":\"RecordBlkView.Signal\",\"uuid\":\"7a3eb810-c178-4b33-8a1f-4ec4e8076906\"},{\"content\":{\"blockPath\":[\"modelo_fisico_OPCUA/Record\"],\"channel\":[1,20],\"dimensions\":[1,32],\"domain\":\"modelo_fisico_opcua/record\",\"lineColor\":\"#4dbeee\",\"parentID\":82,\"plots\":[1],\"port\":4,\"sid\":[],\"signalID\":102,\"signalName\":\"y_perfil\"},\"type\":\"RecordBlkView.Signal\",\"uuid\":\"773da45e-66fe-47bd-a564-c46eab3ad99f\"},{\"content\":{\"blockPath\":[\"modelo_fisico_OPCUA/Record\"],\"channel\":[1,21],\"dimensions\":[1,32],\"domain\":\"modelo_fisico_opcua/record\",\"lineColor\":\"#a2142f\",\"parentID\":82,\"plots\":[],\"port\":4,\"sid\":[],\"signalID\":103,\"signalName\":\"y_perfil\"},\"type\":\"RecordBlkView.Signal\",\"uuid\":\"1dcfc39f-9a11-4080-b0f4-1fc0b58cea96\"},{\"content\":{\"blockPath\":[\"modelo_fisico_OPCUA/Record\"],\"channel\":[1,22],\"dimensions\":[1,32],\"domain\":\"modelo_fisico_opcua/record\",\"lineColor\":\"#139fff\",\"parentID\":82,\"plots\":[],\"port\":4,\"sid\":[],\"signalID\":104,\"signalName\":\"y_perfil\"},\"type\":\"RecordBlkView.Signal\",\"uuid\":\"f55c5bef-511d-42d3-8889-be6042b26dfc\"},{\"content\":{\"blockPath\":[\"modelo_fisico_OPCUA/Record\"],\"channel\":[1,23],\"dimensions\":[1,32],\"domain\":\"modelo_fisico_opcua/record\",\"lineColor\":\"#ff6929\",\"parentID\":82,\"plots\":[],\"port\":4,\"sid\":[],\"signalID\":105,\"signalName\":\"y_perfil\"},\"type\":\"RecordBlkView.Signal\",\"uuid\":\"d588e2e1-5be1-40e5-af04-17a768d86c25\"},{\"content\":{\"blockPath\":[\"modelo_fisico_OPCUA/Record\"],\"channel\":[1,24],\"dimensions\":[1,32],\"domain\":\"modelo_fisico_opcua/record\",\"lineColor\":\"#b746ff\",\"parentID\":82,\"plots\":[],\"port\":4,\"sid\":[],\"signalID\":106,\"signalName\":\"y_perfil\"},\"type\":\"RecordBlkView.Signal\",\"uuid\":\"1561de11-5b82-49d1-9191-95153afd54cd\"},{\"content\":{\"blockPath\":[\"modelo_fisico_OPCUA/Record\"],\"channel\":[1,25],\"dimensions\":[1,32],\"domain\":\"modelo_fisico_opcua/record\",\"lineColor\":\"#64d413\",\"parentID\":82,\"plots\":[],\"port\":4,\"sid\":[],\"signalID\":107,\"signalName\":\"y_perfil\"},\"type\":\"RecordBlkView.Signal\",\"uuid\":\"501b56e5-fd3e-44d6-888f-617d8f2d249b\"},{\"content\":{\"blockPath\":[\"modelo_fisico_OPCUA/Record\"],\"channel\":[1,26],\"dimensions\":[1,32],\"domain\":\"modelo_fisico_opcua/record\",\"lineColor\":\"#ff13a6\",\"parentID\":82,\"plots\":[],\"port\":4,\"sid\":[],\"signalID\":108,\"signalName\":\"y_perfil\"},\"type\":\"RecordBlkView.Signal\",\"uuid\":\"3e59a2a9-a453-4f8e-af2b-13bfae1fb800\"},{\"content\":{\"blockPath\":[\"modelo_fisico_OPCUA/Record\"],\"channel\":[1,27],\"dimensions\":[1,32],\"domain\":\"modelo_fisico_opcua/record\",\"lineColor\":\"#fe330a\",\"parentID\":82,\"plots\":[],\"port\":4,\"sid\":[],\"signalID\":109,\"signalName\":\"y_perfil\"},\"type\":\"RecordBlkView.Signal\",\"uuid\":\"20d970d0-001e-4ddb-9f83-eed95db052ac\"},{\"content\":{\"blockPath\":[\"modelo_fisico_OPCUA/Record\"],\"channel\":[1,28],\"dimensions\":[1,32],\"domain\":\"modelo_fisico_opcua/record\",\"lineColor\":\"#22b573\",\"parentID\":82,\"plots\":[],\"port\":4,\"sid\":[],\"signalID\":110,\"signalName\":\"y_perfil\"},\"type\":\"RecordBlkView.Signal\",\"uuid\":\"171f34ef-737d-4a6b-adf4-5d8f884fe41d\"},{\"content\":{\"blockPath\":[\"modelo_fisico_OPCUA/Record\"],\"channel\":[1,29],\"dimensions\":[1,32],\"domain\":\"modelo_fisico_opcua/record\",\"lineColor\":\"#0072bd\",\"parentID\":82,\"plots\":[],\"port\":4,\"sid\":[],\"signalID\":111,\"signalName\":\"y_perfil\"},\"type\":\"RecordBlkView.Signal\",\"uuid\":\"f3cb6566-f680-4ede-b051-01350acaee5a\"},{\"content\":{\"blockPath\":[\"modelo_fisico_OPCUA/Record\"],\"channel\":[1,30],\"dimensions\":[1,32],\"domain\":\"modelo_fisico_opcua/record\",\"lineColor\":\"#d95319\",\"parentID\":82,\"plots\":[],\"port\":4,\"sid\":[],\"signalID\":112,\"signalName\":\"y_perfil\"},\"type\":\"RecordBlkView.Signal\",\"uuid\":\"e8776949-ef5e-4cff-8faf-37942e886e98\"},{\"content\":{\"blockPath\":[\"modelo_fisico_OPCUA/Record\"],\"channel\":[1,31],\"dimensions\":[1,32],\"domain\":\"modelo_fisico_opcua/record\",\"lineColor\":\"#edb120\",\"parentID\":82,\"plots\":[],\"port\":4,\"sid\":[],\"signalID\":113,\"signalName\":\"y_perfil\"},\"type\":\"RecordBlkView.Signal\",\"uuid\":\"1128a5de-0e88-454c-894a-b4c1c6e755a8\"},{\"content\":{\"blockPath\":[\"modelo_fisico_OPCUA/Record\"],\"channel\":[1,32],\"dimensions\":[1,32],\"domain\":\"modelo_fisico_opcua/record\",\"lineColor\":\"#7e2f8e\",\"parentID\":82,\"plots\":[],\"port\":4,\"sid\":[],\"signalID\":114,\"signalName\":\"y_perfil\"},\"type\":\"RecordBlkView.Signal\",\"uuid\":\"9fc86ab6-6c65-4a13-aef2-e178943432fa\"}]},\"type\":\"RecordBlkView.InputSignals\",\"uuid\":\"5fdf6d25-6721-45dd-a674-a9c5b544710a\"}],\"packageUris\":[\"http://schema.mathworks.com/mf0/streamout_blocks/R2020a\"],\"version\":\"1.0\"}"  VisualizationBindings="{\"xyplotplugin\":{\"info\":[{\"series\":[{\"bindingParametersList\":[{\"parameter\":\"X-Axis\",\"signalID\":9,\"signalName\":\"x_l\"},{\"parameter\":\"Y-Axis\",\"signalID\":12,\"signalName\":\"y_l\"}],\"seriesID\":213},{\"bindingParametersList\":[{\"parameter\":\"X-Axis\",\"signalID\":16,\"signalName\":\"x_perfil(1,1)\"},{\"parameter\":\"Y-Axis\",\"signalID\":83,\"signalName\":\"y_perfil(1,1)\"}],\"seriesID\":320},{\"bindingParametersList\":[{\"parameter\":\"X-Axis\",\"signalID\":17,\"signalName\":\"x_perfil(1,2)\"},{\"parameter\":\"Y-Axis\",\"signalID\":84,\"signalName\":\"y_perfil(1,2)\"}],\"seriesID\":639},{\"bindingParametersList\":[{\"parameter\":\"Y-Axis\",\"signalID\":102,\"signalName\":\"y_perfil(1,20)\"},{\"parameter\":\"X-Axis\",\"signalID\":102,\"signalName\":\"y_perfil(1,20)\"}],\"seriesID\":767}],\"subplotID\":1}]}}"
  Simple : LampBlock  LabelPosition=Hide
  Slider : SliderBlock  ScaleMin=-3  ScaleMax=3  TickInterval=1
  Slider1 : SliderBlock  ScaleMin=-4  ScaleMax=+4  TickInterval=1
  Subsystem : Subsystem
  Twistlocks : LampBlock  LabelPosition=Hide
  Velocidad de Izaje : Scope
  Velocidad de Traslacion : Scope
  "ble   " : LampBlock  LabelPosition=Hide
  carril_fin : Constant  Value=17
  carril_finDoble : Constant  Value=5
  in_carro : Constant  Value=0
  in_izaje : Constant  Value=0
  tag scope: Orden_Nivel0=global, sistOK=global
  wires:
  Modelo Fisico Carro-Izaje-Carga/1(x_td) -> [x_td]
  Modelo Fisico Carro-Izaje-Carga/3(x_hd) -> [x_hd]
  Modelo Fisico Carro-Izaje-Carga/7(theta) -> [theta]
  [yc] -> Modelo Fisico Carro-Izaje-Carga/6(Yc)
  Modelo Fisico Carro-Izaje-Carga/5(x_l) -> [x_l]
  Modelo Fisico Carro-Izaje-Carga/6(y_l) -> [y_l]
  Modelo Fisico Carro-Izaje-Carga/8(F_hw) -> [F_hw]
  Modelo Fisico Carro-Izaje-Carga/2(d_x_td) -> [d_x_td]
  Modelo Fisico Carro-Izaje-Carga/4(d_x_hd) -> [d_x_hd]
  [T_tm] -> Modelo Fisico Carro-Izaje-Carga/2(T_tm)
  [T_hm] -> Modelo Fisico Carro-Izaje-Carga/3(T_hm)
  [ml] -> Modelo Fisico Carro-Izaje-Carga/5(ml)
  [theta] -> Gain3/1  "Angulo de balanceo"
  [F_hw] -> Fuerza de tension del cable/1
  [dx_hd_consigna] -> Mux4/2  "Vel_deseada"
  [d_x_td] -> Mux3/1  "Vel_real"
  [x_hd_consigna] -> Mux2/2  "Pos_deseada"
  Mux2/1 -> Movimiento de Izaje/1
  Mux4/1 -> Velocidad de Izaje/1
  [d_x_hd] -> Mux4/1  "Vel_real"
  [x_td] -> Mux1/1  "Pos_real"
  Mux3/1 -> Velocidad de Traslacion/1
  [x_td_consigna] -> Mux1/2  "Pos_deseada"
  [x_hd] -> Mux2/1  "Pos_real"
  Mux1/1 -> Movimiento de Traslacion/1
  [dx_td_consigna] -> Mux3/2  "Vel_deseada"
  Gain3/1 -> Angulo de balanceo/1
  [BRK_h] -> Modelo Fisico Carro-Izaje-Carga/9(BRK_h)
  [BRK_hE] -> Modelo Fisico Carro-Izaje-Carga/10(BRK_hE)
  [BRK_t] -> Modelo Fisico Carro-Izaje-Carga/8(BRK_t)
  Modelo Fisico Carro-Izaje-Carga/15(fc_inf_ult) -> [fc_inf_ult]
  Modelo Fisico Carro-Izaje-Carga/18(lim_v_h) -> [lim_v_h]
  [cargado] -> Memory5/1
  Memory5/1 -> Modelo Fisico Carro-Izaje-Carga/1(TLK)
  Modelo Fisico Carro-Izaje-Carga/14(fc_inf_norm) -> [fc_inf_norm]
  Modelo Fisico Carro-Izaje-Carga/17(fc_sup_ult) -> [fc_sup_ult]
  Modelo Fisico Carro-Izaje-Carga/13(fc_der_ult) -> [fc_der_ult]
  Modelo Fisico Carro-Izaje-Carga/10(fc_izq_norm) -> [fc_izq_norm]
  Modelo Fisico Carro-Izaje-Carga/11(fc_izq_ult) -> [fc_izq_ult]
  Modelo Fisico Carro-Izaje-Carga/12(fc_der_norm) -> [fc_der_norm]
  Modelo Fisico Carro-Izaje-Carga/16(fc_sup_norm) -> [fc_sup_norm]
  [xc] -> Modelo Fisico Carro-Izaje-Carga/7(Xc)
  [vel_hMax] -> Modelo Fisico Carro-Izaje-Carga/4(vel_hMax)
  [x_l] -> Record/1
  [y_l] -> Record/2
  Modelo Fisico Carro-Izaje-Carga/9(Tension_hw) -> [Tension_hw]
  Estado Final de Frenos/2(BRK_t_def) -> [BRK_t]
  [EMER_H] -> Estado Final de Frenos/6(EMER_h)
  [Orden_Nivel0] -> Estado Final de Frenos/7(Orden_Nivel0)
  Estado Final de Frenos/3(BRK_h_def) -> [BRK_h]
  [EMER_T] -> Estado Final de Frenos/5(EMER_T)
  [sistOK] -> Estado Final de Frenos/4(sistOK)
  Estado Final de Frenos/1(manual_auto_def) -> [manual_auto]
  [ml_medida] -> Nivel 2/2(ml)
  [x_hd] -> Nivel 2/5(x_hd)
  Nivel 2/5(x_td*) -> [x_td_consigna]
  Nivel 2/2(T_tm_on) -> [T_tm_on]
  Nivel 2/4(T_hm_on) -> [T_hm_on]
  [Balanceo_ctrl] -> Nivel 2/1(Balanceo_ctrl)
  Nivel 2/6(x_hd*) -> [x_hd_consigna]
  Nivel 2/8(d_x_hd*) -> [dx_hd_consigna]
  Nivel 2/1(T_tm) -> [T_tm]
  Nivel 2/3(T_hm) -> [T_hm]
  [vel_h] -> Nivel 2/8(vel_h)
  [x_td] -> Nivel 2/4(x_td)
  [in_izaje] -> Nivel 2/6(in_izaje)
  Nivel 2/7(d_x_td*) -> [dx_td_consigna]
  [theta] -> Nivel 2/3(theta)
  [vel_hMax] -> Nivel 2/10(vel_hMax)
  [in_carro] -> Nivel 2/7(in_carro)
  [max_masa] -> Nivel 2/12(max_masa)
  [manual_auto] -> Nivel 2/11(manual_auto)
  [vel_t] -> Nivel 2/9(vel_t)
  [in_carro] -> Compare To Zero7/1
  [in_izaje] -> Compare To Zero2/1
  [T_tm_on] -> Cast To Double17/1
  Demux/8 -> [RESET_OK]
  [T_hm_on] -> Cast To Double18/1
  [fc_izq_ult] -> Cast To Double14/1
  Mux7/1 -> [Orden_Nivel0]
  Demux/3 -> Mux7/2
  [Manual] -> Cast To Double19/1
  [ON_OFF] -> Cast To Double20/1
  Demux/7 -> [EMER_H]
  [lim_v_h] -> Memory12/1
  [BTN_RESET] -> Memory10/1
  [fc_der_ult] -> Cast To Double13/1
  Demux/1 -> [sistOK]
  Demux/4 -> Mux7/3
  [BTN_EMERGENCIA] -> Cast To Double16/1
  Memory12/1 -> Cast To Double15/1
  Demux/2 -> Mux7/1
  Demux/6 -> [EMER_T]
  [fc_inf_ult] -> Cast To Double12/1
  Demux/5 -> [BRK_hE]
  [F_hw] -> Mux/3
  [fc_sup_ult] -> Cast To Double11/1
  Modelo Fisico Carro-Izaje-Carga/19(graficar) -> [graficar]
  Modelo Fisico Carro-Izaje-Carga/20(xc) -> [xc]
  Modelo Fisico Carro-Izaje-Carga/21(yc) -> [yc]
  Modelo Fisico Carro-Izaje-Carga/22(m_l_real) -> [ml]
  Memory10/1 -> Cast To Double10/1
  Constant18/1 -> Manual Switch2/2, Manual Switch4/2, Manual Switch3/2, Manual Switch6/2, Manual Switch7/2, Manual Switch5/2, Manual Switch1/2
  Manual Switch4/1 -> [Balanceo_ctrl]
  in_carro/1 -> [in_carro]
  Manual Switch6/1 -> [BRK_BTN]
  Constant17/1 -> Manual Switch2/1, Manual Switch4/1, Manual Switch3/1, Manual Switch6/1, Manual Switch7/1, Manual Switch5/1, Manual Switch1/1
  Manual Switch1/1 -> [ON_OFF]
  Manual Switch5/1 -> [Ciclo]
  in_izaje/1 -> [in_izaje]
  Manual Switch3/1 -> [TLK]
  Subsystem/1(Out1) -> [BTN_RESET]
  Manual Switch2/1 -> [Manual]
  [RESET_OK] -> Subsystem/1(" ")
  Manual Switch7/1 -> [BTN_EMERGENCIA]
  [BRK_BTN] -> Estado Final de Frenos/8(BRK_BTN)
  Clock/1 -> MATLAB Function1/1(clock)
  [ON_OFF] -> MATLAB Function1/2(ON_OFF)
  [BTN_EMERGENCIA] -> MATLAB Function1/3(BTN_EMERGENCIA)
  [Manual] -> MATLAB Function1/4(Manual)
  [Ciclo] -> MATLAB Function1/5(Ciclo)
  [max_masa] -> MATLAB Function1/6(max_masa)
  [Tension_hw] -> MATLAB Function1/7(Tension_hw)
  [lim_v_h] -> MATLAB Function1/8(lim_v_h)
  [Balanceo] -> MATLAB Function1/9(Balanceo)
  [manual_auto] -> MATLAB Function1/10(manual_auto)
  [ml_medida] -> MATLAB Function1/11(ml_medida)
  [xc] -> MATLAB Function1/12(xc)
  [yc] -> MATLAB Function1/13(yc)
  [graficar] -> MATLAB Function1/14(graficar)
  [x_l] -> MATLAB Function1/15(x_l)
  [y_l] -> MATLAB Function1/16(y_l)
  [x_td] -> MATLAB Function1/17(x_td)
  [manual_auto_1] -> Estado Final de Frenos/1(manual_auto_Nivel1)
  [BRK_t_1] -> Estado Final de Frenos/2(BRK_t)
  [BRK_h_1] -> Estado Final de Frenos/3(BRK_h)
  OPC Read/1 -> Demux/1
  Demux/9 -> [ml_medida]
  Demux/10 -> [vel_t]
  Demux/11 -> [vel_h]
  Demux/12 -> [vel_hMax]
  Demux/13 -> [cargado]
  Demux/14 -> [max_masa]
  Demux/15 -> [Balanceo]
  Demux/16 -> [manual_auto_1]
  Demux/17 -> [BRK_t_1]
  Demux/18 -> [BRK_h_1]
  [Tension_hw] -> Cast To Double7/1
  [d_x_td] -> Mux/18
  [d_x_hd] -> Mux/19
  [x_td] -> Mux/20
  [x_hd] -> Mux/21
  [y_l] -> Mux/23
  [x_l] -> Mux/22
  [fc_izq_norm] -> Cast To Double6/1
  [fc_der_norm] -> Cast To Double5/1
  [fc_inf_norm] -> Cast To Double4/1
  [fc_sup_norm] -> Cast To Double3/1
  [TLK] -> Cast To Double2/1
  [Ciclo] -> Cast To Double1/1
  [Balanceo_ctrl] -> Cast To Double/1
  Mux/1 -> OPC Write/1
  Compare To Zero2/1 -> Cast To Double9/1
  Compare To Zero7/1 -> Cast To Double8/1
  MATLAB Function/1(X_fin) -> Mux/13
  MATLAB Function/2(X_finDoble) -> Mux/14
  carril_fin/1 -> MATLAB Function/1(carrilFin)
  carril_finDoble/1 -> MATLAB Function/2(carrilFinDoble)
  [xc] -> MATLAB Function/3(Xcarga)
  Cast To Double/1 -> Mux/30
  Cast To Double1/1 -> Mux/29
  Cast To Double2/1 -> Mux/28
  Cast To Double3/1 -> Mux/27
  Cast To Double4/1 -> Mux/26
  Cast To Double5/1 -> Mux/25
  Cast To Double6/1 -> Mux/24
  Cast To Double7/1 -> Mux/17
  Cast To Double8/1 -> Mux/16
  Cast To Double9/1 -> Mux/15
  Cast To Double10/1 -> Mux/12
  Cast To Double11/1 -> Mux/11
  Cast To Double12/1 -> Mux/10
  Cast To Double13/1 -> Mux/9
  Cast To Double14/1 -> Mux/8
  Cast To Double15/1 -> Mux/7
  Cast To Double16/1 -> Mux/6
  Cast To Double17/1 -> Mux/5
  Cast To Double18/1 -> Mux/4
  Cast To Double19/1 -> Mux/2
  Cast To Double20/1 -> Mux/1

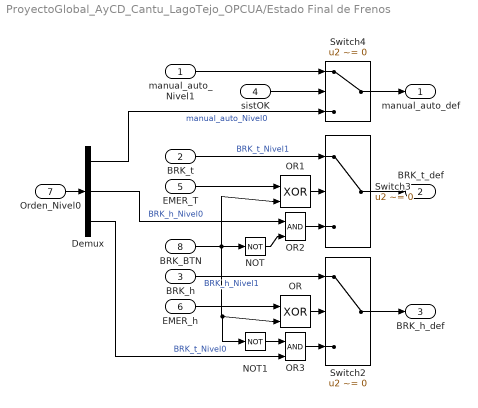
== system ProyectoGlobal_AyCD_Cantu_LagoTejo_OPCUA/Estado Final de Frenos ==
  manual_auto_Nivel1 : Inport
  BRK_t : Inport  Port=2
  BRK_h : Inport  Port=3
  sistOK : Inport  Port=4
  EMER_T : Inport  Port=5
  EMER_h : Inport  Port=6
  Orden_Nivel0 : Inport  Port=7
  BRK_BTN : Inport  Port=8
  Demux : Demux  Outputs=3
  NOT : Logic  Operator=NOT  IconShape=distinctive  AllPortsSameDT=off  OutDataTypeStr=boolean
  NOT1 : Logic  Operator=NOT  IconShape=distinctive  AllPortsSameDT=off  OutDataTypeStr=boolean
  OR : Logic  Operator=XOR  IconShape=distinctive  AllPortsSameDT=off  OutDataTypeStr=boolean
  OR1 : Logic  Operator=XOR  IconShape=distinctive  AllPortsSameDT=off  OutDataTypeStr=boolean
  OR2 : Logic  IconShape=distinctive  AllPortsSameDT=off  OutDataTypeStr=boolean
  OR3 : Logic  IconShape=distinctive  AllPortsSameDT=off  OutDataTypeStr=boolean
  Switch2 : Switch  Criteria=u2 ~= 0
  Switch3 : Switch  Criteria=u2 ~= 0
  Switch4 : Switch  Criteria=u2 ~= 0
  manual_auto_def : Outport
  BRK_t_def : Outport  Port=2
  BRK_h_def : Outport  Port=3
  wires:
  Switch3/1 -> BRK_t_def/1
  Switch2/1 -> BRK_h_def/1
  Switch4/1 -> manual_auto_def/1
  sistOK/1 -> Switch4/2
  BRK_t/1 -> Switch3/1  "BRK_t_Nivel1"
  BRK_h/1 -> Switch2/1  "BRK_h_Nivel1"
  manual_auto_Nivel1/1 -> Switch4/1
  Demux/2 -> OR2/1  "BRK_h_Nivel0"
  Demux/3 -> OR3/2  "BRK_t_Nivel0"
  Orden_Nivel0/1 -> Demux/1
  Demux/1 -> Switch4/3  "manual_auto_Nivel0"
  OR/1 -> Switch2/2
  EMER_T/1 -> OR1/1
  OR1/1 -> Switch3/2
  BRK_BTN/1 -> OR1/2, NOT/1, NOT1/1, OR/2
  OR2/1 -> Switch3/3
  NOT/1 -> OR2/2
  EMER_h/1 -> OR/1
  OR3/1 -> Switch2/3
  NOT1/1 -> OR3/1
